simulink model "Sixteen_PSK"  (R2017a)
settings: Solver=VariableStepAuto  StartTime=0.0  StopTime=10.0  RelTol=1e-3
undefined symbols (not defined in the file or in its folder): comm, constellation
libraries: commdigbbndpm3 x2, commchan3 x1, commutil2 x1, commsink2 x1, commrflib2 x1, commrandsrc3 x1
settings Model: Creator=sarriola  LastModifiedBy=sarriola

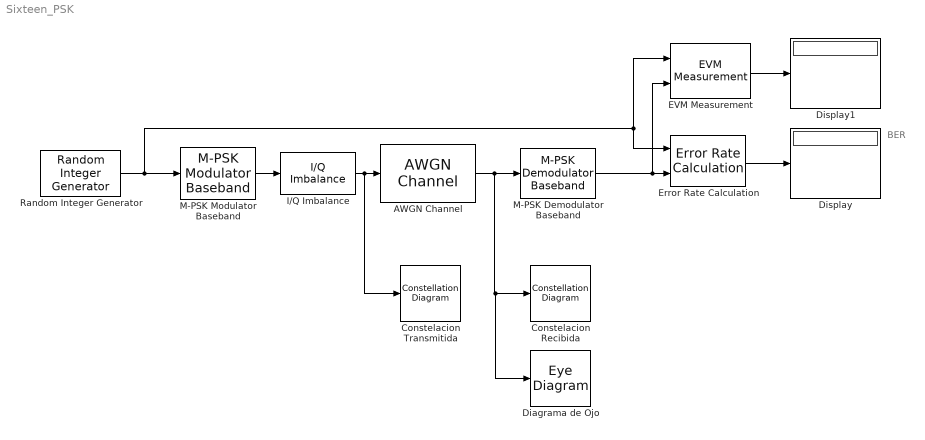
== system Sixteen_PSK ==
  note: BER
  AWGN Channel : commchan3/AWGN Channel  InputProcessing=Columns as channels (frame based)  seed=67  noiseMode="Signal to noise ratio  (SNR)"  EbNodB=10  EsNodB=10  SNRdB=-5  bitsPerSym=3  Ps=1  Tsym=1e-6  variance=1
  "Constelacion Recibida " : ConstellationDiagram
  Constelacion Transmitida : ConstellationDiagram
  "Diagrama de Ojo " : EyeDiagram
  Display : Display
  Display1 : Display
  EVM Measurement : commutil2/EVM Measurement  Normalization=Average reference signal power  AverageConstellationPower=1  PeakConstellationPower=1  ReferenceSignalSource=Input port  ReferenceConstellation=constellation( comm.QPSKModulator )  MeasurementIntervalSource=Input length  MeasurementInterval=100  AveragingDimensions=1  MaximumEVMOutputPort=off  XPercentileEVMOutputPort=off  XPercentileValue=95  SymbolCountOutputPort=off  SimulateUsing=Interpreted execution
      settings: SourceProductName=Communications System Toolbox  SourceProductBaseCode=CM
  Error Rate Calculation : commsink2/Error Rate Calculation  N=0  st_delay=0  cp_mode=Entire frame  subframe=[]  PMode=Port  WsName=ErrorVec  RsMode2=off  stop=off  numErr=100  maxBits=1e6
  I/Q Imbalance : commrflib2/I//Q Imbalance  ampImbal=-10  phsImbal=45  Idc=0  Qdc=0
      settings: SourceProductName=Communications System Toolbox  SourceProductBaseCode=CM
  M-PSK Demodulator Baseband : commdigbbndpm3/M-PSK Demodulator Baseband  M=16  OutType=Integer  DecType=Hard decision  VarSource=Dialog  Variance=1  Dec=Gray  Mapping=[0:7]  Ph=0  outDtype1=Inherit via internal rule  outDtype2=Inherit via internal rule  derotateFactorWordLen=16  derotateFactorDataTypeStr=Inherit: Same word length as input  derotateFactorLastDataTypeStr=Inherit: Same word length as input
      settings: SourceProductName=Communications System Toolbox
  M-PSK Modulator Baseband : commdigbbndpm3/M-PSK Modulator Baseband  M=16  InType=Integer  Enc=Gray  Mapping=[0:7]  Ph=0  outDtype=double  outWordLen=16  outUDDataType=sfix(16)  outFracLenMode=Best precision  outFracLen=15  outDataTypeStr=double  outLastDataTypeStr=double
      settings: SourceProductName=Communications System Toolbox
  Random Integer Generator : commrandsrc3/Random Integer Generator  SetSize=16  SeedSource=Auto  Seed=0  SampleTime=1e-6  SamplesPerFrame=1024  OutputDataType=double  SimulateUsing=Interpreted execution
  wires:
  EVM Measurement/1 -> Display1/1
  AWGN Channel/1 -> "Diagrama de Ojo "/1, "Constelacion Recibida "/1, M-PSK Demodulator Baseband/1
  Error Rate Calculation/1 -> Display/1
  M-PSK Demodulator Baseband/1 -> EVM Measurement/2, Error Rate Calculation/2
  Random Integer Generator/1 -> M-PSK Modulator Baseband/1, EVM Measurement/1, Error Rate Calculation/1
  M-PSK Modulator Baseband/1 -> I/Q Imbalance/1
  I/Q Imbalance/1 -> Constelacion Transmitida/1, AWGN Channel/1
